simulink model "discrete_controller"  (R2018a)
settings: Solver=VariableStepAuto  StartTime=0.0  StopTime=10.0  RelTol=1e-3
undefined symbols (not defined in the file): Cd2_den, Cd2_num, G_den, G_num, reference, T
settings Model: Creator=julio  LastModifiedBy=julio

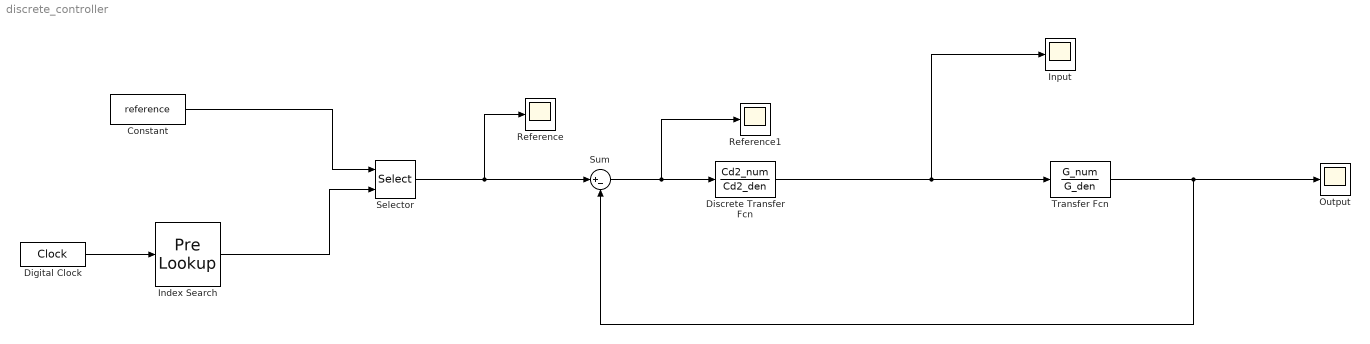
== system discrete_controller ==
  Constant : Constant  Value=reference
  Digital Clock : DigitalClock  SampleTime=T
  Discrete Transfer Fcn : DiscreteTransferFcn  Numerator=Cd2_num  Denominator=Cd2_den  SampleTime=T
  Index Search : PreLookup  BreakpointsData=time  OutputSelection=Index only
  Input : Scope
  Output : Scope
  Reference : Scope
  Reference1 : Scope
  Selector : Selector  IndexMode=Zero-based  IndexOptions=Index vector (port)  Indices=[1 3]  OutputSizes=1
  Sum : Sum  Inputs=|+-
  Transfer Fcn : TransferFcn  Numerator=G_num  Denominator=G_den
  wires:
  Transfer Fcn/1 -> Output/1, Sum/2
  Discrete Transfer Fcn/1 -> Input/1, Transfer Fcn/1
  Selector/1 -> Reference/1, Sum/1
  Sum/1 -> Reference1/1, Discrete Transfer Fcn/1
  Digital Clock/1 -> Index Search/1
  Constant/1 -> Selector/1
  Index Search/1 -> Selector/2
